simulink model "MotorXploer"  (R2025a)
settings: Solver=FixedStepAuto  StartTime=0.0  StopTime=inf  FixedStep=0.001  RelTol=1e-3
undefined symbols (not defined in the file or in its folder): Blocking, LF, Non
libraries: dspstat3 x4, amg_usbconverter_n_connect_lib x3
settings Model: Creator=beamk  LastModifiedBy=ACER

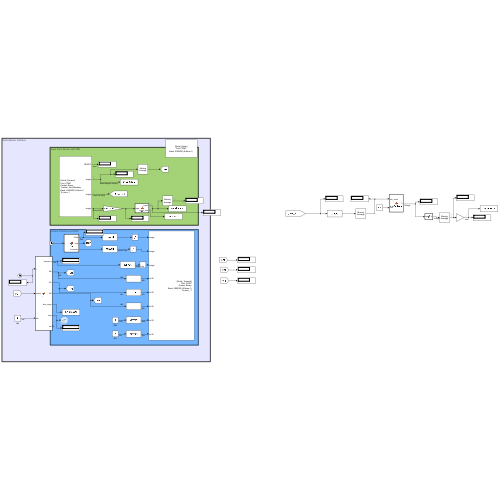
[thumbnail: Simulink's stored preview of the top-level diagram]
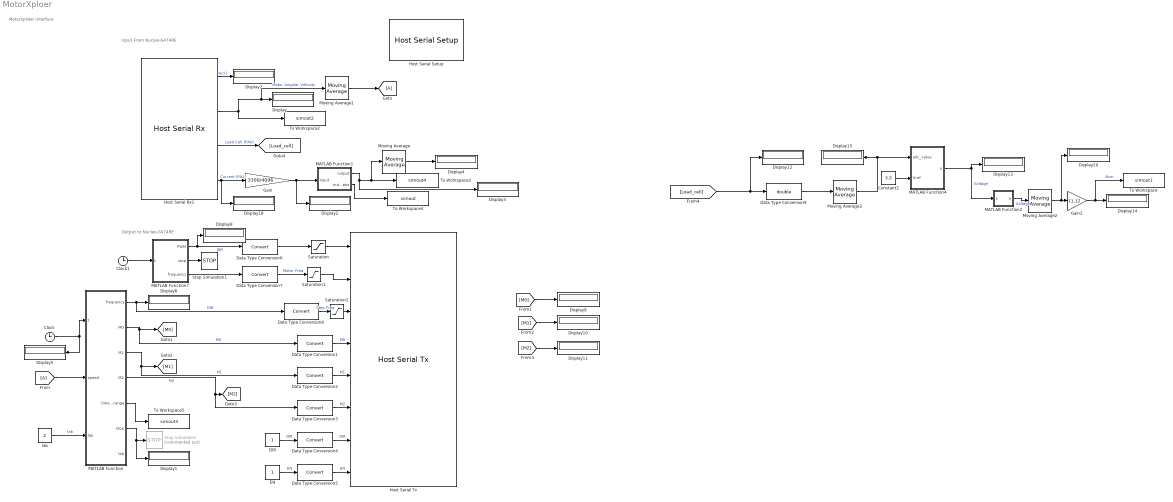
== system MotorXploer ==
  note: Output to Nucleo-G474RE
  note: Input From Nucleo-G474RE
  note: MotorXploler Interface
  Clock : Clock
  Clock1 : Clock
  Constant2 : Constant  Value=3.3
  DIR : Constant
  Data Type Conversion{1..8} (8 alike) : DataTypeConversion  SaturateOnIntegerOverflow=off  RndMeth=Floor
  Data Type Conversion9 : DataTypeConversion  OutDataTypeStr=double  SaturateOnIntegerOverflow=off  RndMeth=Floor
  Display{,1..15,18,20} (18 alike) : Display
  EN : Constant
  From : From
  Gain : Gain  Gain=3300/4096
  Gain2 : Gain  Gain=11.12
  Goto : Goto
  Host Serial Rx1 : amg_usbconverter_n_connect_lib/Host Serial Rx  conf=rx  port=<auto>  baudrate=2000000  databits=8  parity=None  stopbit=1  flowcontrol=None  transfer=Non-Blocking  timeout=5  packetmode=Binary  enableinitialvalues=off  initialvalues=[]  binheader='25'  binterminator='4E'  porttype_double=0  porttype_single=3  porttype_int8=0  porttype_uint8=0  porttype_int16=0  porttype_uint16=0  porttype_int32=0  porttype_uint32=0  asciiformat='%f,%f,%d,%d'  rx_asciiterminator="LF (0x0A - \"\\n\")"  tx_asciiterminator="CRLF (0x0D 0x0A - \"\\r\\n\")"  sampletime=-1  enablecustomportlabel=off  cinputportlabel=0  coutputportlabel=A  portpinstr=0  blockid=HostSerialRx1  inputporttype=[]  inputportwidth=[]  inputportlabel={}  outputporttype=[3 1 1 1]  outputportwidth=[1 1 1 1]  outputportlabel={'READY','single','single','single'}  compat=0  optionstring=[]  autoport='COM7'
  Host Serial Setup : amg_usbconverter_n_connect_lib/Host Serial Setup  conf=setup  port=<auto>  baudrate=2000000  databits=8  parity=None  stopbit=1  flowcontrol=None  transfer=Blocking  timeout=2  packetmode=Binary  initialvalues=[]  binheader='7E 7E'  binterminator='03 03'  porttype_double=0  porttype_single=1  porttype_int8=0  porttype_uint8=0  porttype_int16=0  porttype_uint16=0  porttype_int32=0  porttype_uint32=2  asciiformat='%d %u %x'  rx_asciiterminator="CRLF (0x0D 0x0A - \"\\r\\n\")"  tx_asciiterminator="CRLF (0x0D 0x0A - \"\\r\\n\")"  sampletime=-1  enablecustomportlabel=off  cinputportlabel=0  coutputportlabel=A  portpinstr=0  blockid=HostSerialSetup  inputporttype=[]  inputportwidth=[]  inputportlabel={}  outputporttype=[]  outputportwidth=[]  outputportlabel={}  compat=0  optionstring=[]  autoport='COM7'
  Host Serial Tx : amg_usbconverter_n_connect_lib/Host Serial Tx  conf=tx  port=<auto>  baudrate=2000000  databits=8  parity=None  stopbit=1  flowcontrol=None  transfer=Blocking  timeout=2  packetmode=Binary  initialvalues=[]  binheader='25'  binterminator='4E'  porttype_double=0  porttype_single=3  porttype_int8=0  porttype_uint8=0  porttype_int16=5  porttype_uint16=0  porttype_int32=0  porttype_uint32=0  asciiformat='%d,%f'  rx_asciiterminator="CRLF (0x0D 0x0A - \"\\r\\n\")"  tx_asciiterminator="CRLF (0x0D 0x0A - \"\\r\\n\")"  sampletime=-1  enablecustomportlabel=off  cinputportlabel=0  coutputportlabel=A  portpinstr=0  blockid=HostSerialTx  inputporttype=[1 1 1 4 4 4 4 4]  inputportwidth=[1 1 1 1 1 1 1 1]  inputportlabel={'single','single','single','int16','int16','int16','int16','int16'}  outputporttype=[]  outputportwidth=[]  outputportlabel={}  compat=0  optionstring=[]  autoport='COM7'
      settings: SourceProductName=aMG USB Converter N
  MATLAB Function : MATLAB Function  TreatAsAtomicUnit=on
  MATLAB Function1 : MATLAB Function  TreatAsAtomicUnit=on
  MATLAB Function2 : MATLAB Function  TreatAsAtomicUnit=on
  MATLAB Function4 : MATLAB Function  TreatAsAtomicUnit=on
  MATLAB Function7 : MATLAB Function  TreatAsAtomicUnit=on
  Moving Average : dspstat3/Moving Average  Method=Exponential weighting  ForgettingFactorPort=off  SpecifyWindowLength=on  WindowLength=4  OverlapLength=3  AllowArbitraryInputLength=off  ForgettingFactor=1  SimulateUsing=Interpreted execution
  Moving Average1 : dspstat3/Moving Average  Method=Exponential weighting  ForgettingFactorPort=off  SpecifyWindowLength=on  WindowLength=4  OverlapLength=3  AllowArbitraryInputLength=off  ForgettingFactor=0.95  SimulateUsing=Interpreted execution
  Moving Average2 : dspstat3/Moving Average  Method=Sliding window  ForgettingFactorPort=off  SpecifyWindowLength=on  WindowLength=4  OverlapLength=3  AllowArbitraryInputLength=off  ForgettingFactor=0.95  SimulateUsing=Interpreted execution
  Moving Average3 : dspstat3/Moving Average  Method=Sliding window  ForgettingFactorPort=off  SpecifyWindowLength=on  WindowLength=4  OverlapLength=3  AllowArbitraryInputLength=off  ForgettingFactor=0.9  SimulateUsing=Interpreted execution
  Saturation : Saturate  UpperLimit=65535  LowerLimit=-65535
  Saturation1 : Saturate  UpperLimit=20000  LowerLimit=0
  Saturation2 : Saturate  UpperLimit=inf  LowerLimit=0
  Stop Simulation : Stop  Commented=on
  Stop Simulation1 : Stop
  To Workspace : ToWorkspace  VariableName=simout1  SaveFormat=Structure With Time  SampleTime=-1
  To Workspace2 : ToWorkspace  VariableName=simout2  SaveFormat=Structure With Time  SampleTime=-1
  To Workspace3 : ToWorkspace  VariableName=simout4  SaveFormat=Structure With Time  SampleTime=-1
  To Workspace4 : ToWorkspace  VariableName=simout  SaveFormat=Structure With Time  SampleTime=-1
  To Workspace5 : ToWorkspace  VariableName=simout3  SaveFormat=Structure With Time  SampleTime=-1
  lab : Constant  Value=2
  wires:
  Host Serial Rx1/2 -> Moving Average1/1, Display/1, To Workspace2/1  "Motor Angular Velocity"
  MATLAB Function/2(M0) -> Data Type Conversion1/1, [M0]  "M0"
  EN/1 -> Data Type Conversion5/1  "EN"
  DIR/1 -> Data Type Conversion4/1  "DIR"
  MATLAB Function/3(M1) -> Data Type Conversion2/1, [M1]  "M1"
  MATLAB Function/4(M2) -> Data Type Conversion3/1, [M2]  "M2"
  MATLAB Function7/3(frequency) -> Data Type Conversion7/1
  Data Type Conversion1/1 -> Host Serial Tx/4  "M0"
  Data Type Conversion2/1 -> Host Serial Tx/5  "M1"
  Data Type Conversion3/1 -> Host Serial Tx/6  "M2"
  Data Type Conversion4/1 -> Host Serial Tx/7  "DIR"
  Data Type Conversion5/1 -> Host Serial Tx/8  "EN"
  Data Type Conversion6/1 -> Saturation/1
  Saturation/1 -> Host Serial Tx/1
  Data Type Conversion7/1 -> Saturation1/1  "Motor Freq"
  Data Type Conversion8/1 -> Saturation2/1  "Step Freq"
  Saturation1/1 -> Host Serial Tx/2
  Saturation2/1 -> Host Serial Tx/3
  Host Serial Rx1/4 -> Gain/1, Display18/1  "Current (PA1)"
  Gain/1 -> Display2/1, MATLAB Function1/1(input)
  MATLAB Function1/1(output) -> Moving Average/1, To Workspace3/1, Display3/1
  Host Serial Rx1/1 -> Display7/1  "wcs1"
  Moving Average/1 -> Display4/1
  MATLAB Function1/2(output_abs) -> To Workspace4/1
  Clock/1 -> Display5/1, MATLAB Function/1(t)
  Moving Average1/1 -> Goto/1
  MATLAB Function/5(time_range) -> To Workspace5/1
  [M0] -> Display9/1
  [M1] -> Display10/1
  [M2] -> Display11/1
  [Load_cell] -> Data Type Conversion9/1, Display12/1
  Constant2/1 -> MATLAB Function4/2(Vref)
  Moving Average2/1 -> Display20/1, Gain2/1
  Data Type Conversion9/1 -> Moving Average3/1
  Gain2/1 -> To Workspace/1, Display14/1  "Ncm"
  Moving Average3/1 -> MATLAB Function4/1(adc_value), Display15/1
  MATLAB Function4/1(V) -> Display13/1, MATLAB Function2/1(input)  "Voltage"
  Host Serial Rx1/3 -> [Load_cell]  "Load Cell (PA0)"
  MATLAB Function/1(frequency) -> Data Type Conversion8/1, Display6/1  "DIR"
  From/1 -> MATLAB Function/2(speed)
  lab/1 -> MATLAB Function/3("lab ")  "lab"
  MATLAB Function/6(stop) -> Display1/1, Stop Simulation/1
  MATLAB Function7/1(PWM) -> Display8/1, Data Type Conversion6/1  "DIR"
  Clock1/1 -> MATLAB Function7/1(t)
  MATLAB Function7/2(stop) -> Stop Simulation1/1
  MATLAB Function2/1(V) -> Moving Average2/1  "Voltage"

== matlab function MotorXploer/MATLAB Function1 ==
  data: input input; output output; output_abs output
function [output,output_abs] = fcn(input)

output = (input - 2890)/27;
output_abs = abs(input - 1704)/27;

== matlab function MotorXploer/MATLAB Function ==
  data: t input; frequency output; M0 output; M1 output; M2 output; time_range output; speed input; stop output; lab output; lab input
function [frequency, M0, M1, M2, time_range, stop, lab] = fcn(t, speed, lab)
%#codegen

persistent cycleStartTime
detectDelay = 40;        % detect 0-speed AFTER this time (case 1)
frequency_stop = 6000;   % target stop frequency for case 2

% Initialize
if isempty(cycleStartTime)
    cycleStartTime = 0;
end

% Defaults
M0 = 0; M1 = 0; M2 = 0;
frequency = 0;
stop = 0;

dt = t - cycleStartTime;
time_range = [cycleStartTime t];

switch lab

    % ============================================================
    % CASE 1 : Your original logic
    % ============================================================
    case 1

        if dt < 3
            frequency = 900;
            return;
        end

        block = floor(dt - 3) + 1;
        if block < 1
            block = 1;
        end

        frequency = block * 50;

        if dt < detectDelay
            return;
        end

        if speed <= 1
            frequency = 0;
            stop = 1;
        end


    % ============================================================
    % CASE 2 : Same ramp as Case 1, but stop at frequency_stop
    % ============================================================
    case 2
        
        % Before dt = 3 sec → fixed 900 Hz (same as case 1)


        % Same ramp block logic as case 1
        block = floor(t) + 1;
        if block < 1
            block = 1;
        end

        frequency = block * 50;

        % Stop when reaching frequency_stop
        if frequency >= frequency_stop
            frequency = 0;
            stop = 1;
        end


    % ============================================================
    % DEFAULT (safety)
    % ============================================================
    otherwise
        frequency = 0;
        stop = 1;
end

end

== matlab function MotorXploer/MATLAB Function2 ==
  data: input input; V output
function V = kg(input)
    V = (input-1.37)*1289.74;
end

== matlab function MotorXploer/MATLAB Function4 ==
  data: adc_value input; V output; Vref input
function V = adc2voltage(adc_value, Vref)
    % ตรวจสอบขอบเขตค่าของ ADC
    if any(adc_value < 0 | adc_value > 4095)
        error('adc_value range 0 - 4095');
    end

    % คำนวณแรงดัน
    V = (adc_value / 4095) * Vref;
end

== matlab function MotorXploer/MATLAB Function7 ==
  data: t input; PWM output; stop output; frequency output
function [PWM, stop, frequency] = fcn(t)
%#codegen

frequency = 50;      % constant frequency
stop = 0;            % default value

% PWM ramp from 0 → 65536 as time goes 0 → 100
PWM = (floor(t)/100 *5*65536);
% PWM = 0;

% When t reaches exactly 100 → stop
if PWM >= 65536
    stop = 1;
    PWM = 0;     % optional: clamp PWM to max
end

end
